simulink model "EISGov_SelectTrqLim"  (R2016b)
settings: configuration reference "CodeGenConfigSet" (kept outside this file)
values from neighbouring files (symbols this model uses):
  EISGov_trqRedHiLimMin_C = Calibration.Parameter    [init_EISGov_SelectTrqLim.m]    (also in init_EISGov_SelectTrqLim_SIL.m = Simulink.Parameter)
  TRQ_ZERO = fi(0,Trq_Nm)    [init_EISGov_SelectTrqLim.m]    (also in init_EISGov_SelectTrqLim_SIL.m)
undefined symbols (not defined in the file or in its folder): EISGov_num_conv
libraries: simulink x4
settings Model: Creator=Administrator  LastModifiedBy=liutao
settings ConfigSetRef: SourceLocation=Base Workspace

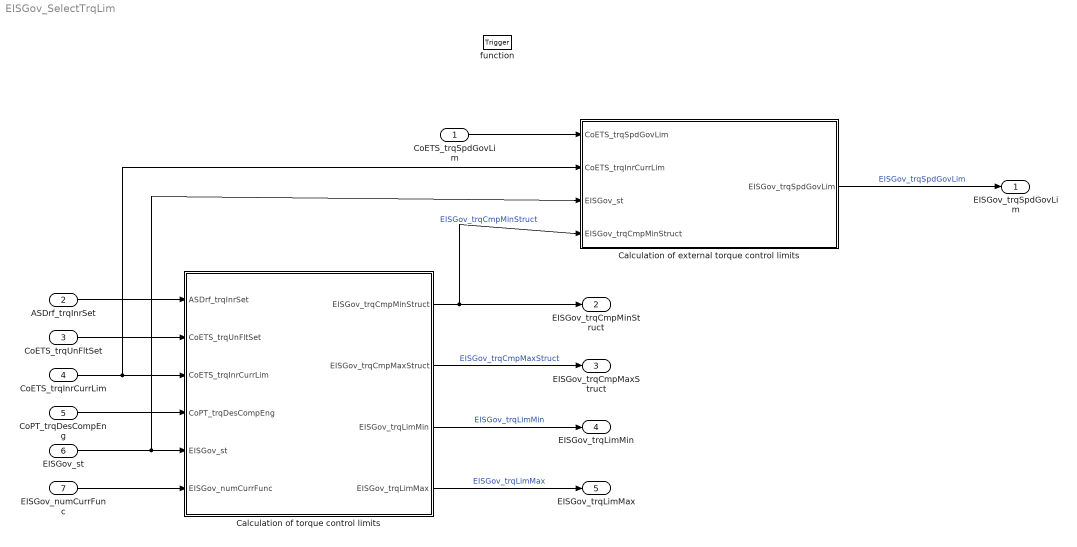
== system EISGov_SelectTrqLim ==
  CoETS_trqSpdGovLim : Inport  Tag=Nm  Description=Inner engine limitation torque for EISGov  OutMin=-3276.8  OutMax=3276.7  OutDataTypeStr=Trq_Nm
  ASDrf_trqInrSet : Inport  Tag=Nm  Description=ASD reference filter torque output  Port=2  OutMin=-3000  OutMax=3000  OutDataTypeStr=Trq_Nm
  CoETS_trqUnFltSet : Inport  Tag=Nm  Description="Compensation torque of \"loss torque compensation\" to bypass filter influences on the set path which is partly compensated"  Port=3  OutMin=-3276  OutMax=3276  OutDataTypeStr=Trq_Nm
  CoETS_trqInrCurrLim : Inport  Tag=Nm  Description=Current lowest limitation torque (inner engine torque)  Port=4  OutMin=-3276.8  OutMax=3276.7  OutDataTypeStr=Trq_Nm
  CoPT_trqDesCompEng : Inport  Tag=Nm  Description=Application parameter for engine torque desired for compensation  Port=5  OutMin=-3276  OutMax=3276  OutDataTypeStr=Trq_Nm
  EISGov_st : Inport  Description=Status information of EISGov and its clients  Port=6  OutMin=0  OutMax=2147483648  OutDataTypeStr=State_uint32
  EISGov_numCurrFunc : Inport  Description=Identification name / number of the currently active EISGov client, which determines the current controller parameters  Port=7  OutDataTypeStr=Enum: EISGov_num_conv
  function : TriggerPort  TriggerType=function-call  VariantControl=Variant
  Calculation of external torque control limits : Subsystem
  Calculation of torque control limits : Subsystem
  EISGov_trqSpdGovLim : Outport  Tag=Nm  Description=limitation for inner engine torque  OutMin=-3276.8  OutMax=3276.7  OutDataTypeStr=Trq_Nm
  EISGov_trqCmpMinStruct : Outport  Tag=Nm  Description=Torque limitation of the controlling torque path (relevant in case of MIN structure)  Port=2  OutMin=-3276.8  OutMax=3276.7  OutDataTypeStr=Trq_Nm
  EISGov_trqCmpMaxStruct : Outport  Tag=Nm  Description=Torque limitation of the controlling torque path (relevant in case of MAX structure)  Port=3  OutMin=-3276.8  OutMax=3276.7  OutDataTypeStr=Trq_Nm
  EISGov_trqLimMin : Outport  Tag=Nm  Description=lower torque control limit for EISGov  Port=4  OutMin=-3276.8  OutMax=3276.7  OutDataTypeStr=Trq_Nm
  EISGov_trqLimMax : Outport  Tag=Nm  Description=Upper torque control limit for EISGov  Port=5  OutMin=-3276.8  OutMax=3276.7  OutDataTypeStr=Trq_Nm
  wires:
  CoETS_trqInrCurrLim/1 -> Calculation of torque control limits/3(CoETS_trqInrCurrLim), Calculation of external torque control limits/2(CoETS_trqInrCurrLim)
  ASDrf_trqInrSet/1 -> Calculation of torque control limits/1(ASDrf_trqInrSet)
  CoETS_trqUnFltSet/1 -> Calculation of torque control limits/2(CoETS_trqUnFltSet)
  CoPT_trqDesCompEng/1 -> Calculation of torque control limits/4(CoPT_trqDesCompEng)
  EISGov_numCurrFunc/1 -> Calculation of torque control limits/6(EISGov_numCurrFunc)
  Calculation of torque control limits/1(EISGov_trqCmpMinStruct) -> EISGov_trqCmpMinStruct/1, Calculation of external torque control limits/4(EISGov_trqCmpMinStruct)  "EISGov_trqCmpMinStruct"
  EISGov_st/1 -> Calculation of torque control limits/5(EISGov_st), Calculation of external torque control limits/3(EISGov_st)
  Calculation of torque control limits/4(EISGov_trqLimMax) -> EISGov_trqLimMax/1  "EISGov_trqLimMax"
  Calculation of torque control limits/2(EISGov_trqCmpMaxStruct) -> EISGov_trqCmpMaxStruct/1  "EISGov_trqCmpMaxStruct"
  Calculation of torque control limits/3(EISGov_trqLimMin) -> EISGov_trqLimMin/1  "EISGov_trqLimMin"
  CoETS_trqSpdGovLim/1 -> Calculation of external torque control limits/1(CoETS_trqSpdGovLim)
  Calculation of external torque control limits/1(EISGov_trqSpdGovLim) -> EISGov_trqSpdGovLim/1  "EISGov_trqSpdGovLim"

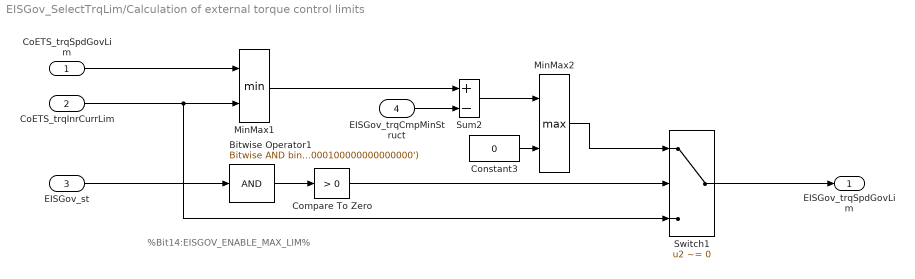
== system EISGov_SelectTrqLim/Calculation of external torque control limits ==
  note: %Bit14:EISGOV_ENABLE_MAX_LIM%
  CoETS_trqSpdGovLim : Inport
  CoETS_trqInrCurrLim : Inport  Port=2
  EISGov_st : Inport  Port=3
  EISGov_trqCmpMinStruct : Inport  Port=4
  Bitwise Operator1 : simulink/Logic and Bit Operations/Bitwise Operator  logicop=AND  UseBitMask=on  BitMask=bin2dec('00000000000000000100000000000000')  BitMaskRealWorld=Stored Integer
  Compare To Zero : simulink/Logic and Bit Operations/Compare To Zero  relop=>  OutDataTypeStr=boolean
  Constant3 : Constant  Value=0  OutDataTypeStr=Inherit: Inherit via back propagation
  MinMax1 : MinMax  Inputs=2
  MinMax2 : MinMax  Function=max  Inputs=2  InputSameDT=on
  Sum2 : Sum  Inputs=+-  SaturateOnIntegerOverflow=on  InputSameDT=on
  Switch1 : Switch  Criteria=u2 ~= 0
  EISGov_trqSpdGovLim : Outport
  wires:
  CoETS_trqInrCurrLim/1 -> MinMax1/2, Switch1/3
  EISGov_st/1 -> Bitwise Operator1/1
  EISGov_trqCmpMinStruct/1 -> Sum2/2
  MinMax2/1 -> Switch1/1
  MinMax1/1 -> Sum2/1
  CoETS_trqSpdGovLim/1 -> MinMax1/1
  Switch1/1 -> EISGov_trqSpdGovLim/1
  Sum2/1 -> MinMax2/1
  Constant3/1 -> MinMax2/2
  Bitwise Operator1/1 -> Compare To Zero/1
  Compare To Zero/1 -> Switch1/2

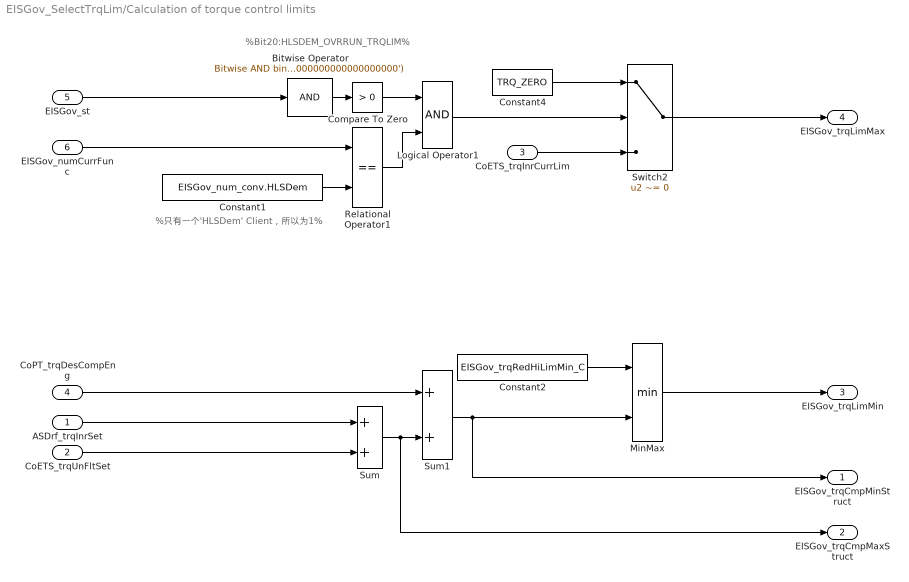
== system EISGov_SelectTrqLim/Calculation of torque control limits ==
  note: %只有一个'HLSDem' Client，所以为1%
  note: %Bit20:HLSDEM_OVRRUN_TRQLIM%
  ASDrf_trqInrSet : Inport
  CoETS_trqUnFltSet : Inport  Port=2
  CoETS_trqInrCurrLim : Inport  Port=3
  CoPT_trqDesCompEng : Inport  Port=4
  EISGov_st : Inport  Port=5
  EISGov_numCurrFunc : Inport  Port=6
  Bitwise Operator : simulink/Logic and Bit Operations/Bitwise Operator  logicop=AND  UseBitMask=on  BitMask=bin2dec('00000000000100000000000000000000')  BitMaskRealWorld=Stored Integer
  Compare To Zero : simulink/Logic and Bit Operations/Compare To Zero  relop=>  OutDataTypeStr=boolean
  Constant1 : Constant  Value=EISGov_num_conv.HLSDem
  Constant2 : Constant  Value=EISGov_trqRedHiLimMin_C
  Constant4 : Constant  Value=TRQ_ZERO  OutDataTypeStr=Trq_Nm
  Logical Operator1 : Logic  AllPortsSameDT=off  OutDataTypeStr=boolean
  MinMax : MinMax  Inputs=2  InputSameDT=on
  Relational Operator1 : RelationalOperator  Operator===  OutDataTypeStr=boolean  RndMeth=Nearest  InputSameDT=on
  Sum : Sum  SaturateOnIntegerOverflow=on  InputSameDT=on
  Sum1 : Sum  SaturateOnIntegerOverflow=on  InputSameDT=on
  Switch2 : Switch  Criteria=u2 ~= 0  InputSameDT=on
  EISGov_trqCmpMinStruct : Outport
  EISGov_trqCmpMaxStruct : Outport  Port=2
  EISGov_trqLimMin : Outport  Port=3
  EISGov_trqLimMax : Outport  Port=4
  wires:
  Constant2/1 -> MinMax/1
  Switch2/1 -> EISGov_trqLimMax/1
  Relational Operator1/1 -> Logical Operator1/2
  Bitwise Operator/1 -> Compare To Zero/1
  EISGov_numCurrFunc/1 -> Relational Operator1/1
  CoETS_trqInrCurrLim/1 -> Switch2/3
  EISGov_st/1 -> Bitwise Operator/1
  CoETS_trqUnFltSet/1 -> Sum/2
  Logical Operator1/1 -> Switch2/2
  Sum1/1 -> EISGov_trqCmpMinStruct/1, MinMax/2
  Constant4/1 -> Switch2/1
  CoPT_trqDesCompEng/1 -> Sum1/1
  ASDrf_trqInrSet/1 -> Sum/1
  Constant1/1 -> Relational Operator1/2
  MinMax/1 -> EISGov_trqLimMin/1
  Sum/1 -> Sum1/2, EISGov_trqCmpMaxStruct/1
  Compare To Zero/1 -> Logical Operator1/1
